simulink model "imu_gait_detection"  (R2019b)
settings: Solver=ode5  StartTime=0.0  StopTime=10.0  FixedStep=0.002  RelTol=1e-3  EnableMultiTasking=on
model workspace (MAT data in the model file):
  can_receive_message_id = 1409
  can_send_message_id = 1409
undefined symbols (not defined in the file or in its folder): CAN_Device, PEAK, sldrtexcb_modeswitch, System
libraries: sldrtlib x6, canmsglib x4, simulink x3
Description:
  | CAN Input/Output with Vehicle Network Toolbox
  | 
  | The example model "sldrtex_canmessage" shows how to transfer data through CAN bus, utilizing the
  | CAN_MESSAGE data type and the CAN Pack and CAN Unpack blocks available
  | in Vehicle Network Toolbox block library. The CAN_MESSAGE data type can
  | be directly processed by Simulink Desktop Real-Time blocks.
  | The model sends data within one computer, from one CAN channel to another.
  | The two CAN channels can be either virtual channels or physical channels
  | on a dual-channel CAN device. You can modify the
  | model to communicate between two computers by splitting this model
  | into its send and receive parts and running the models on two computers.
  | The yellow blocks are used to send the data, the blue blocks
  | are used to receive the data.
  | 
  | How to run this model in Normal Mode:
  | 
  | 1) Double-click the orange button to switch to Normal Mode if needed.
  | 2) Start the real-time execution using Simulation->Run.
  | 
  | How to run this model in External Mode:
  | 
  | 1) Double-click the orange button to switch to External Mode if needed.
  | 2) Double-click the orange button to switch to External Mode if needed.
  | 3) Start the real-time execution using Simulation->Run. The model will automatically
  |    build, connect to Simulink in External Mode and start.
  | 
  | Note: This model runs on Microsoft Windows only.
settings Model: SimulationMode=external  ExtModeTrigDuration=1001  OrderedModelArguments=off  Creator=The MathWorks, Inc.  LastModifiedBy=wumin
settings DataIOCC: MaxDataPoints=100000  SaveFormat=Array  SaveOutput=off  SignalLogging=off  DSMLogging=off  SaveTime=off  ReturnWorkspaceOutputs=off
settings OptimizationCC: MemcpyThreshold=1024  ExpressionDepthLimit=2147483647  InitFltsAndDblsToZero=on  EfficientMapNaN2IntZero=off
settings DebuggingCC: UnderspecifiedInitializationDetection=Classic  MergeDetectMultiDrivingBlocksExec=none  SolverPrmCheckMsg=warning  FcnCallInpInsideContextMsg=warning  AllowSymbolicDim=off  StateNameClashWarn=warning  SFUnexpectedBacktrackingDiag=warning  SFNoUnconditionalDefaultTransitionDiag=warning  SFExecutionAtInitializationDiag=none  ArithmeticOperatorsInVariantConditions=warning
settings HardwareCC: TargetBitPerLong=64  TargetBitPerPointer=64  TargetBitPerSizeT=64  TargetBitPerPtrDiffT=64  TargetIntDivRoundTo=Zero  TargetEndianess=LittleEndian  TargetWordSize=64  TargetHWDeviceType=Intel->x86-64
settings ModelReferenceCC: PropagateSignalLabelsOutOfModel=off
settings SFSimCC: SimUseLocalCustomCode=off
settings RTWCC: Description=Simulink Desktop Real-Time  SystemTargetFile=sldrt.tlc  TemplateMakefile=sldrt.tmf  RTWUseLocalCustomCode=off  RTWCompilerOptimization=on
settings CodeAppCC: MaxIdLength=95  StateflowObjectComments=on
settings SimulinkDesktopRealTimeCC: TargetPreCompLibLocation=D:\Matlab2019b\toolbox\sldrt\lib\win64  TargetLangStandard=C89/C90 (ANSI)  PreserveStateflowLocalDataDimensions=off
settings ConfigComp: CovMetricSettings=dw  CovHtmlReporting=on  CovSaveCumulativeToWorkspaceVar=on  CovSaveSingleToWorkspaceVar=on  CovShowResultsExplorer=off  CovExternalEMLEnable=off  CovSFcnEnable=off

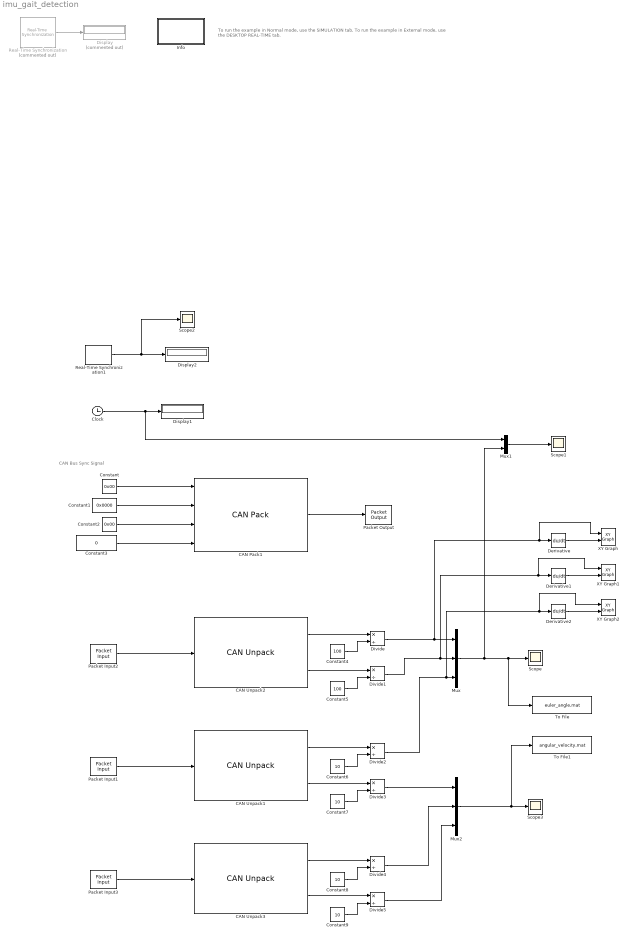
== system imu_gait_detection ==
  note: CAN Bus Sync Signal
  note: To run the example in Normal mode, use the SIMULATION tab.
      | To run the example in External mode, use the DESKTOP REAL-TIME tab.
  CAN Pack1 : canmsglib/CAN Pack  MsgList=(none)  MsgName=CANopen Msg  MsgIDType=Standard (11-bit identifier)  MsgIdentifier=0x80  MsgLength=8  Remote=off  ApplyMinMax=off  BusOutput=off  SignalInfo={ 'Operation', '0', '8', 'LE', 'unsigned', 'Standard', '0', '1', '0', '-Inf', 'Inf'; 'Index', '8', '16', 'LE', 'unsigned', 'Standard', '0', '1', '0', '-Inf', 'Inf'; 'SubIndex', '24', '8', 'LE', 'unsigned', 'Standard', '0', '1', '0', '-Inf', 'Inf'; 'Data', '32', '32', 'LE', 'unsigned', 'Standard', '0', '1', '0', '-Inf', 'Inf' }
      settings: SourceProductName=Vehicle Network Toolbox  SourceProductBaseCode=VN  DataFormat=manually specified signals
  CAN Unpack1 : canmsglib/CAN Unpack  MsgList=(none)  MsgName=CANopen Msg  MsgIDType=Standard (11-bit identifier)  MsgIdentifier=0x281  MsgLength=8  SignalInfo={ 'EulerAngleZ', '0', '32', 'LE', 'signed', 'Standard', '0', '1', '0', '-Inf', 'Inf'; 'AngularVelocityX', '32', '32', 'LE', 'signed', 'Standard', '0', '1', '0', '-Inf', 'Inf' }  IDPort=off  TimestampPort=off  ErrorPort=off  RemotePort=off  LengthPort=off  StatusPort=off  ApplyMinMax=off
      settings: SourceProductName=Vehicle Network Toolbox  SourceProductBaseCode=VN
  CAN Unpack2 : canmsglib/CAN Unpack  MsgList=(none)  MsgName=CANopen Msg  MsgIDType=Standard (11-bit identifier)  MsgIdentifier=0x181  MsgLength=8  SignalInfo={ 'EulerAngleX', '0', '32', 'LE', 'signed', 'Standard', '0', '1', '0', '-Inf', 'Inf'; 'EulerAngleY', '32', '32', 'LE', 'signed', 'Standard', '0', '1', '0', '-Inf', 'Inf' }  IDPort=off  TimestampPort=off  ErrorPort=off  RemotePort=off  LengthPort=off  StatusPort=off  ApplyMinMax=off
      settings: SourceProductName=Vehicle Network Toolbox  SourceProductBaseCode=VN
  CAN Unpack3 : canmsglib/CAN Unpack  MsgList=(none)  MsgName=CANopen Msg  MsgIDType=Standard (11-bit identifier)  MsgIdentifier=0x381  MsgLength=8  SignalInfo={ 'AngularVelocityY', '0', '32', 'LE', 'signed', 'Standard', '0', '1', '0', '-Inf', 'Inf'; 'AngularVelocityZ', '32', '32', 'LE', 'signed', 'Standard', '0', '1', '0', '-Inf', 'Inf' }  IDPort=off  TimestampPort=off  ErrorPort=off  RemotePort=off  LengthPort=off  StatusPort=off  ApplyMinMax=off
      settings: SourceProductName=Vehicle Network Toolbox  SourceProductBaseCode=VN
  Clock : Clock
  Constant : Constant  Value=0x00  OutDataTypeStr=uint8  SampleTime=0
  Constant1 : Constant  Value=0x0000  OutDataTypeStr=uint16
  Constant2 : Constant  Value=0x00  OutDataTypeStr=uint8
  Constant3 : Constant  Value=0  OutDataTypeStr=uint32
  Constant4 : Constant  Value=100
  Constant5 : Constant  Value=100
  Constant{6..9} (4 alike) : Constant  Value=10
  Derivative : Derivative
  Derivative1 : Derivative
  Derivative2 : Derivative
  Display : Display  Commented=on
  Display1 : Display
  Display2 : Display
  Divide{,1..5} (6 alike) : Product  Inputs=*/
  Info : Subsystem  InitFcn=sldrtexcb_modeswitch('CheckKernel');  mask(Simulink Desktop Real-Time Example Info){}
      settings: OpenFcn=helpview([docroot '/sldrt/helptargets.map'], 'CANInputOutputWithVNTExample')
      mask Display: disp('Info')
  Mux : Mux  Inputs=3
  Mux1 : Mux  Inputs=2
  Mux2 : Mux  Inputs=3
  Packet Input1 : sldrtlib/Packet Input  SampleTime=-1  MaxMissedTicks=1000  ShowMissedTicks=off  YieldWhenWaiting=off  DrvName=PEAK-System/CAN_Device  DrvAddress=81  DrvOptions=[0 0 0 0 1000]  PacketSize=8  DataTypes='CAN_MESSAGE'  ShowReady=off  ShowError=off  PacketID=2048e0 + (double(0x281))  ByteOrder=1  ShowTimestamp=off
      settings: AttributesFormatString=PEAK-System\nCAN Device [81]  SourceProductName=Simulink Desktop Real-Time
  Packet Input2 : sldrtlib/Packet Input  SampleTime=-1  MaxMissedTicks=1000  ShowMissedTicks=off  YieldWhenWaiting=off  DrvName=PEAK-System/CAN_Device  DrvAddress=81  DrvOptions=[0 0 0 0 1000]  PacketSize=8  DataTypes='CAN_MESSAGE'  ShowReady=off  ShowError=off  PacketID=2048e0 + (double(0x181))  ByteOrder=1  ShowTimestamp=off
      settings: AttributesFormatString=PEAK-System\nCAN Device [81]  SourceProductName=Simulink Desktop Real-Time
  Packet Input3 : sldrtlib/Packet Input  SampleTime=-1  MaxMissedTicks=1000  ShowMissedTicks=off  YieldWhenWaiting=off  DrvName=PEAK-System/CAN_Device  DrvAddress=81  DrvOptions=[0 0 0 0 1000]  PacketSize=8  DataTypes='CAN_MESSAGE'  ShowReady=off  ShowError=off  PacketID=2048e0 + (double(0x381))  ByteOrder=1  ShowTimestamp=off
      settings: AttributesFormatString=PEAK-System\nCAN Device [81]  SourceProductName=Simulink Desktop Real-Time
  Packet Output : sldrtlib/Packet Output  SampleTime=-1  MaxMissedTicks=1000  ShowMissedTicks=off  YieldWhenWaiting=off  DrvName=PEAK-System/CAN_Device  DrvAddress=81  DrvOptions=[0 0 0 0 1000]  PacketSize=8  DataTypes='CAN_MESSAGE'  ShowReady=off  ShowError=off  PacketID=2048e0 + (double(0x80))  ByteOrder=1  InitialValue=[]  FinalValue=[]
      settings: AttributesFormatString=PEAK-System\nCAN Device [81]  SourceProductName=Simulink Desktop Real-Time
  Real-Time Synchronization : sldrtlib/Real-Time Synchronization  Commented=on  SampleTime=0.01  MaxMissedTicks=10  ShowMissedTicks=on  YieldWhenWaiting=off
  Real-Time Synchronization1 : sldrtlib/Real-Time Synchronization  SampleTime=-1  MaxMissedTicks=1000  ShowMissedTicks=on  YieldWhenWaiting=off
  Scope{,1..3} (4 alike) : Scope
  To File : ToFile  Filename=euler_angle.mat  SaveFormat=Timeseries
  To File1 : ToFile  Filename=angular_velocity.mat  SaveFormat=Timeseries
  XY Graph : simulink/Sinks/XY Graph  xmin=-100  xmax=100  ymin=-100  ymax=100  st=-1
  XY Graph1 : simulink/Sinks/XY Graph  xmin=-100  xmax=100  ymin=-100  ymax=100  st=-1
  XY Graph2 : simulink/Sinks/XY Graph  xmin=-100  xmax=100  ymin=-100  ymax=100  st=-1
  wires:
  Real-Time Synchronization/1 -> Display/1
  Clock/1 -> Mux1/1, Display1/1
  Constant1/1 -> CAN Pack1/2
  Constant3/1 -> CAN Pack1/4
  Constant2/1 -> CAN Pack1/3
  Constant/1 -> CAN Pack1/1
  CAN Pack1/1 -> Packet Output/1
  Packet Input2/1 -> CAN Unpack2/1
  Packet Input1/1 -> CAN Unpack1/1
  CAN Unpack2/1 -> Divide/1
  CAN Unpack2/2 -> Divide1/1
  CAN Unpack1/1 -> Divide2/1
  Divide/1 -> XY Graph/1, Derivative/1, Mux/1
  Constant4/1 -> Divide/2
  Constant5/1 -> Divide1/2
  Constant6/1 -> Divide2/2
  Mux/1 -> Mux1/2, To File/1, Scope/1
  Mux1/1 -> Scope1/1
  Real-Time Synchronization1/1 -> Scope2/1, Display2/1
  Packet Input3/1 -> CAN Unpack3/1
  Constant7/1 -> Divide3/2
  CAN Unpack1/2 -> Divide3/1
  Constant8/1 -> Divide4/2
  CAN Unpack3/1 -> Divide4/1
  Constant9/1 -> Divide5/2
  CAN Unpack3/2 -> Divide5/1
  Divide3/1 -> Mux2/1
  Divide4/1 -> Mux2/2
  Divide5/1 -> Mux2/3
  Mux2/1 -> To File1/1, Scope3/1
  Derivative/1 -> XY Graph/2
  Divide1/1 -> XY Graph1/1, Derivative1/1, Mux/2
  Derivative1/1 -> XY Graph1/2
  Divide2/1 -> XY Graph2/1, Derivative2/1, Mux/3
  Derivative2/1 -> XY Graph2/2

== system imu_gait_detection/Info ==
